simulink model "sqlite_adclogging_demo"  (Simulink 7.3)
settings: Solver=FixedStepDiscrete  SolverMode=SingleTasking  StartTime=0.0  StopTime=10.0  RelTol=1e-3
PreLoadFcn:
  | waijung.modelPreload; % Required for working with Waijung Blockset. Do not remove.
undefined symbols (not defined in the file): Blocking, HSEOSC, Link, LQFP176, Non, ST, STM32F417IG
libraries: amg_sqlite_dataserver x3, simulink x1, stm32f4_adc_lib x1, stm32f4_device_config_lib x1
CloseFcn:
  | waijung.modelClose; % Required for working with Waijung Blockset. Do not remove.
settings Model: Creator=Krisada  LastModifiedBy=Krisada
settings OptimizationCC: OptimizeModelRefInitCode=on  LifeSpan=1
settings HardwareCC: ProdEndianess=LittleEndian  ProdHWDeviceType=ARM Compatible->Cortex - M4  TargetEndianess=LittleEndian  TargetHWDeviceType=ARM Compatible->Cortex - M4
settings RTWCC: SystemTargetFile=stm32f4.tlc  GenerateMakefile=off  TemplateMakefile=ert_default_tmf  Description=STM32F4 Target  ProcessScript=stm32f4_make_rtw_hook
settings CodeAppCC: IgnoreCustomStorageClasses=off
settings STFCustomTargetCC: ModelReferenceCompliant=off  CombineOutputUpdateFcns=on  ERTCustomFileBanners=on  SupportContinuousTime=off  SupportNonInlinedSFcns=off  SystemTargetFile=stm32f4.tlc
settings ERTTargetCC: MultiwordLength=2048  ModelReferenceCompliant=off  ParMdlRefBuildCompliant=off  CompOptLevelCompliant=off  ERTFirstTimeCompliant=off  ModelStepFunctionPrototypeControlCompliant=off  CPPClassGenCompliant=off  ExtModeMexFile=noextcomm  InlinedParameterPlacement=NonHierarchical  ERTSrcFileBannerTemplate=stm32f4_code_template.cgt  ERTHdrFileBannerTemplate=stm32f4_code_template.cgt  ERTDataSrcFileTemplate=stm32f4_code_template.cgt  ERTDataHdrFileTemplate=stm32f4_code_template.cgt  ERTCustomFileTemplate=stm32f4_file_process.tlc

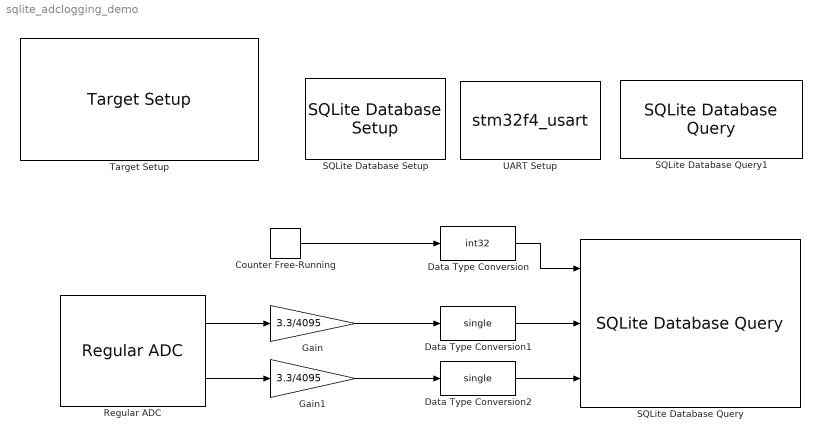
== system sqlite_adclogging_demo ==
  Counter Free-Running : simulink/Sources/Counter Free-Running  SystemSampleTime=-1  NumBits=32  tsamp=-1
  Data Type Conversion : DataTypeConversion  OutDataTypeMode=int32  OutDataType=fixdt(1, 16)  OutScaling=2^0  OutDataTypeStr=int32
  Data Type Conversion1 : DataTypeConversion  OutDataTypeMode=single  OutDataType=fixdt(1, 16)  OutScaling=2^0  OutDataTypeStr=single
  Data Type Conversion2 : DataTypeConversion  OutDataTypeMode=single  OutDataType=fixdt(1, 16)  OutScaling=2^0  OutDataTypeStr=single
  Gain : Gain  Gain=3.3/4095  ParameterDataType=fixdt(1, 16)  ParameterScaling=2^0  OutDataType=fixdt(1, 16)  OutScaling=2^0
  Gain1 : Gain  Gain=3.3/4095  ParameterDataType=fixdt(1, 16)  ParameterScaling=2^0  OutDataType=fixdt(1, 16)  OutScaling=2^0
  Regular ADC : stm32f4_adc_lib/Regular ADC  adcmodule=1  outputdatatype=Double  prescaler=2  prescalerstr=ADC_Prescaler_Div2  chsamplingtime=Auto  chsamplingtimestr=ADC_SampleTime_480Cycles  read_an0=off  read_an1=off  read_an2=off  read_an3=off  read_an4=off  read_an5=off  read_an6=off  read_an7=off  read_an8=off  read_an9=off  read_an10=off  read_an11=off  read_an12=off  read_an13=off  read_an14=on  read_an15=on  read_an16=off  read_an17=off  read_an18=off  pinstr=GPIO_Pin_14 | GPIO_Pin_15  usedpinarray="[0  0  0  0  0  0  0  0  0  0  0  0  0  0  1  1  0  0  0]"  usedportidarray="[2  2]"  usedpinidarray="[4  5]"  usedpinidcount=2  sampletime=0.001  blockid=RegularADC  enablecustomportlabel=off  cinputportlabel=0  coutputportlabel=Out1, Out2
  SQLite Database Query : amg_sqlite_dataserver/SQLite Database Query  Priority=1  transfer=Non-Blocking  statement=INSERT  filenameoption=Specific  filename='database.db'  tablenameoption=Specific  tablename='sensors'  columns='id integer, adc1 real, adc2 real'  condition='where rowid==1'  preview=INSERT INTO %s (id,adc1,adc2)VALUES(%d,%f,%f);  enablestatus=off  columncount=3  columnnamesarray="[\"id\",\"adc1\",\"adc2\"]"  columntypesarray="[\"int32\",\"single\",\"single\"]"  inputtypearray=[6 1 1]  outputtypearray=[]  sampletime=-1  sampletimestr=0.001  blockid=SQLiteDatabaseQuery
  SQLite Database Query1 : amg_sqlite_dataserver/SQLite Database Query  Priority=1  transfer=Non-Blocking  statement=CREATE  filenameoption=Specific  filename='database.db'  tablenameoption=Specific  tablename='sensors'  columns='id integer, adc1 real, adc2 real'  condition='where rowid==1'  preview=CREATE TABLE IF NOT EXISTS %s(id integer, adc1 real, adc2 real);  enablestatus=off  columncount=3  columnnamesarray="[\"id\",\"adc1\",\"adc2\"]"  columntypesarray="[\"int32\",\"single\",\"single\"]"  inputtypearray=[]  outputtypearray=[]  sampletime=inf  sampletimestr=0.001  blockid=SQLiteDatabaseQuery1
  SQLite Database Setup : amg_sqlite_dataserver/SQLite Database Setup  Priority=1  port=UART6  timeout=5  buffersize=4096  reset=Software  resetport=A  resetpin=0  inputtypearray=[0]  outputtypearray=[0]  sampletime=inf  sampletimestr=0.001  blockid=SQLiteDatabaseSetup
  Target Setup : stm32f4_device_config_lib/Target Setup  Priority=100  compiler=GNU ARM  previous_compiler=GNU ARM  mcu=STM32F417IG (LQFP176)  mcustr=STM32F417IG  clockconfig=HSEOSC-8MHz  system_stm32f4xx_c_path=F:\trunk\targets\stm32f4_target\stm32f4\utils\system_stm32f4xx_default\STM32F40_41xxx\hseosc8mhz  showmemoryconfiguration=off  stacksize=0x400  heapsize=0x200  enableautocompiledownload=on  fullchiperase=off  programmerinterface=ST-Link  editctrlstr=on  compilercontrolstr=$(patsubst %, -I%, .) -mcpu=cortex-m4 -mthumb -mthumb-interwork -mfloat-abi=hard -mfpu=fpv4-sp-d16 -ffast-math -Wall -Wextra -Ofast  assemblercontrolstr=$(patsubst %, -I%, .) -mcpu=cortex-m4 -mthumb -mthumb-interwork -mfloat-abi=hard -mfpu=fpv4-sp-d16 -ffast-math -Wall -Wextra -Ofast -Wa,-amhls=$(<:.s=.lst) -D__STACK_SIZE=$(STACK_SIZE) -D__HEAP_SIZE=$(HEAP_SIZE)  linkercontrolstr=-T$(LD_SCRIPT) -g -Wl,-Map=$(MAP),--cref,--no-warn-mismatch -mcpu=cortex-m4 -mthumb -mthumb-interwork -mfloat-abi=hard -mfpu=fpv4-sp-d16 -specs=nosys.specs  runafterdownload=on  execprofile=None  profileruart=1  profilerbaud=115200  profilertxpin=D8  profilerinitstr=0.001,168000000,168000,115200,0  manualsetsampletime=off  sampletime=0.001  blockid=TargetSetup  systickreloadvalue=168000  hseval=8000000  lastprofileruart=1  hclk=168000000  flashorigin=0x8000000  flashlength=1024k  ramorigin=0x20000000  ramlength=128k  useextram=off
  UART Setup : S-Function  Priority=1  FunctionName=stm32f4_usart  Parameters=configuration,uartmodule,transfer,baudrate,inputtype,outputtype,confstr,binheaderarray,binterminatorarray,asciiheader,asciiterminator,bindatalength,packetmode,varname,sampletime,sampletimestr,blockid  EnableBusSupport=off  mask(stm32f4_usart){configuration=Setup, uartmodule=6, baudrate=1000000, databits=8, parity=No, stopbit=1, remaptxpin=C6, remaprxpin=C7, flowcontrol=None, remapctspin=Not used, remaprtspin=Not used, advanceoptions=on, rxbuffersize=1024, txbuffersize=1024, transfer=Blocking, packetmode=Ascii, binheader='7E 7E', binterminator='03 03', porttype_double=1, porttype_single=0, porttype_int8=1, porttype_uint8=0, porttype_int16=0, porttype_uint16=0, porttype_int32=0, porttype_uint32=0, asciiformat='%d,%f', rx_asciiterminator=CRLF (0x0D 0x0A - "\r\n"), tx_asciiterminator=CR (0x0D - "\r"), storagename=<empty>, varname=, inputtype=[0], outputtype=[0], binheaderarray=[0], binterminatorarray=[0], bindatalength=0, asciiheader='', asciiterminator=[0], sampletime=-1, sampletimestr=0.001, blockid=UARTSetup, confstr=[ "dummy", "1", "C", "6", "1", "C", "7", "0", "*", "*", "0", "*", "*", "2", "5", "6", "2", "5", "1", "1024", "1024", "2", "6", "1000000", "8", "No", "1", "None", "USART6"], lastmodule=6}
      mask prompts: uartmodule "UART Module"; baudrate "Baud rate (bps)"; databits "Data bits"; stopbit "Stop bit"; remaptxpin "Tx Pin"; remaprxpin "Rx Pin"; flowcontrol "Hardware flow control"; remapctspin "HW Flow control, CTS Pin"; remaprtspin "HW Flow control, RTS Pin"; advanceoptions "Advance options"; rxbuffersize "Rx buffer size (bytes)"; txbuffersize "Tx buffer size (bytes)"; packetmode "Packet mode"; binheader "Binary header (example: '7E 7E')"; binterminator "Binary terminator (example: '03 03')"; porttype_double "Number of data port, type DOUBLE"; porttype_single "Number of data port, type SINGLE"; porttype_int8 "Number of data port, type INT8"; porttype_uint8 "Number of data port, type UINT8"; porttype_int16 "Number of data port, type INT16"; porttype_uint16 "Number of data port, type UINT16"; porttype_int32 "Number of data port, type INT32"; porttype_uint32 "Number of data port, type UINT32"; asciiformat "Ascii format"; rx_asciiterminator "End of packet"; tx_asciiterminator "End of packet"; storagename "Buffer"; varname "Var name"; inputtype "Input data type"; outputtype "Output data type"; binheaderarray "Binary header"; binterminatorarray "Binary terminator"; bindatalength "Binary data length"; asciiheader "Ascii header (printf format)"; asciiterminator "Ascii terminator"; sampletime "Sample time (sec)"; sampletimestr "Compiled sample time (sec) in string"; confstr "Configuration string"; lastmodule "Last module selected"
      mask init:
      | stm32f4_usart_callback('init');
      mask Help: web(fullfile(waijungdocroot,'stm32f4_usart_setup.htm'), '-browser')
      mask StyleString: popup(Setup|Tx|Rx),popup(1|2|3|4|5|6),edit,popup(8),popup(No|Odd|Even),popup(0.5|1|1.5|2),popup(Not used|C6|G14),popup(Not used|C7|G9),popup(None|RTS|CTS|RTS/CTS),popup(Not used|G13|G15),popup(Not used|G8|G12),checkbox,popup(16|32|64|128|256|512|1024|2048),popup(16|32|64|128|256|512|1024|2048),popup(Blocking|Non-Blocking),popup(Ascii|Binary|String Buffer),edit,edit,edit,edit,edit,edit,edit,edit,edit,edit,edit,popup(CR (0x0D - "\r")|LF (0x0A - "\n")|CRLF (0x0D 0x0A - "\r\n")),popup(CR (0x0D - "\r")|LF (0x0A - "\n")|CRLF (0x0D 0x0A - "\r\n")|None),popup(<empty>),edit,edit,edit,edit,edit,edit,edit,edit,edit,edit,edit,edit,edit
      mask CallbackString: stm32f4_usart_callback('configuration');|stm32f4_usart_callback('uartmodule');|stm32f4_usart_callback('baudrate');||||||stm32f4_usart_callback('flowcontrol');|||stm32f4_usart_callback('advanceoptions');|||stm32f4_usart_callback('transfer');|stm32f4_usart_callback('packetmode');|stm32f4_usart_callback('binheader');|stm32f4_usart_callback('binterminator');|stm32f4_usart_callback('porttype');|stm32f4_usart_callback('porttype');|stm32f4_usart_callback('porttype');|stm32f4_usart_callback('porttype');|stm32f4_usart_callback('porttype');|stm32f4_usart_callback('porttype');|stm32f4_usart_callback('porttype');|stm32f4_usart_callback('porttype');|stm32f4_usart_callback('asciiformat');|stm32f4_usart_callback('rx_asciiterminator');|stm32f4_usart_callback('tx_asciiterminator');|stm32f4_usart_callback('storagename');|stm32f4_usart_callback('varname');||||||||stm32f4_usart_callback('sampletime');|stm32f4_usart_callback('sampletimestr');|stm32f4_usart_callback('blockid');||
      mask Display: text(0.5, 0.5, 'Module: USART6_Setup\nBaud (Bps): 1000000\nDMA Buffer: 1024/1024\nTx/Rx Pin: C6/C7','ver','middle','hor','center');
  wires:
  Regular ADC/1 -> Gain/1
  Gain/1 -> Data Type Conversion1/1
  Regular ADC/2 -> Gain1/1
  Gain1/1 -> Data Type Conversion2/1
  Counter Free-Running/1 -> Data Type Conversion/1
  Data Type Conversion/1 -> SQLite Database Query/1
  Data Type Conversion1/1 -> SQLite Database Query/2
  Data Type Conversion2/1 -> SQLite Database Query/3
